simulink model "bf16_mac_new"  (R2022b)
settings: Solver=VariableStepAuto  StartTime=0.0  StopTime=10.0  RelTol=1e-3
libraries: hdlsllib x116, simulink x24
(part 2 of 2)

== system bf16_mac_new/bf16_adder/leading 2 ==
  u : Inport
  MATLAB Function : MATLAB Function  TreatAsAtomicUnit=on
  y : Outport
  wires:
  u/1 -> MATLAB Function/1(u)
  MATLAB Function/1(y) -> y/1

== system bf16_mac_new/bf16_adder/shift left1 ==
  In1 : Inport
  In2 : Inport  Port=2
  Constant : Constant  Value=2  OutDataTypeStr=half
  Data Type Conversion1 : DataTypeConversion  OutDataTypeStr=uint8  SaturateOnIntegerOverflow=off  RndMeth=Floor
  Data Type Conversion2 : DataTypeConversion  OutDataTypeStr=half  SaturateOnIntegerOverflow=off  RndMeth=Floor
  Pow : Math  Operator=pow  SignedPower=on  RndMeth=Zero
  Product : Product
  Out1 : Outport
  wires:
  Pow/1 -> Data Type Conversion1/1
  Constant/1 -> Pow/1
  In2/1 -> Data Type Conversion2/1
  Product/1 -> Out1/1
  Data Type Conversion1/1 -> Product/2
  Data Type Conversion2/1 -> Pow/2
  In1/1 -> Product/1

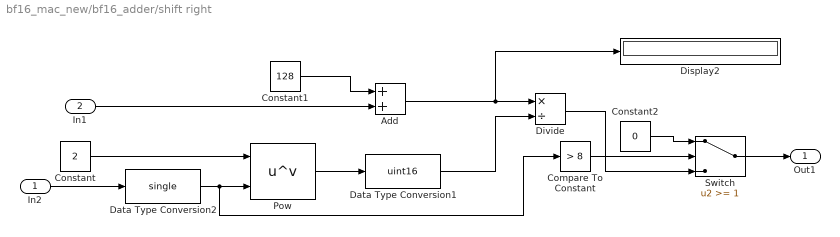
== system bf16_mac_new/bf16_adder/shift right ==
  In2 : Inport
  In1 : Inport  Port=2
  Add : Sum
  Compare To Constant : simulink/Logic and Bit Operations/Compare To Constant  relop=>  const=8  OutDataTypeStr=boolean
  Constant : Constant  Value=2  OutDataTypeStr=single
  Constant1 : Constant  Value=128  OutDataTypeStr=uint8
  Constant2 : Constant  Value=0  OutDataTypeStr=uint8
  Data Type Conversion1 : DataTypeConversion  OutDataTypeStr=uint16  SaturateOnIntegerOverflow=off  RndMeth=Floor
  Data Type Conversion2 : DataTypeConversion  OutDataTypeStr=single  SaturateOnIntegerOverflow=off  RndMeth=Floor
  Display2 : Display
      settings: Format=binary (Stored Integer)
  Divide : Product  Inputs=*/
  Pow : Math  Operator=pow  SignedPower=on  RndMeth=Zero
  Switch : Switch  Threshold=1  SaturateOnIntegerOverflow=off  InputSameDT=off
  Out1 : Outport
  wires:
  Pow/1 -> Data Type Conversion1/1
  Constant/1 -> Pow/1
  In2/1 -> Data Type Conversion2/1
  Data Type Conversion1/1 -> Divide/2
  Data Type Conversion2/1 -> Compare To Constant/1, Pow/2
  Add/1 -> Display2/1, Divide/1
  In1/1 -> Add/2
  Constant1/1 -> Add/1
  Compare To Constant/1 -> Switch/2
  Constant2/1 -> Switch/1
  Divide/1 -> Switch/3
  Switch/1 -> Out1/1

== system bf16_mac_new/bf16_adder/Multiplication1/bit slice ==
  Input : Inport
  Display : Display
      settings: Format=binary (Stored Integer)
  Extract Exponent : hdlsllib/Logic and Bit Operations/Bit Slice  lidx=14  ridx=7
  Extract Mantissa : hdlsllib/Logic and Bit Operations/Bit Slice  lidx=6  ridx=0
  Extract Sign : hdlsllib/Logic and Bit Operations/Bit Slice  lidx=15  ridx=15
  S1 : Outport
  E1 : Outport  Port=2
  M1 : Outport  Port=3
  wires:
  Input/1 -> Extract Mantissa/1, Extract Exponent/1, Extract Sign/1, Display/1
  Extract Mantissa/1 -> M1/1  "mantissa"
  Extract Sign/1 -> S1/1  "sign"
  Extract Exponent/1 -> E1/1

== system bf16_mac_new/bf16_adder/Multiplication1/bit slice1 ==
  Input : Inport
  Display : Display
      settings: Format=binary (Stored Integer)
  Extract Exponent : hdlsllib/Logic and Bit Operations/Bit Slice  lidx=14  ridx=7
  Extract Mantissa : hdlsllib/Logic and Bit Operations/Bit Slice  lidx=6  ridx=0
  Extract Sign : hdlsllib/Logic and Bit Operations/Bit Slice  lidx=15  ridx=15
  S2 : Outport
  E2 : Outport  Port=2
  M2 : Outport  Port=3
  wires:
  Input/1 -> Extract Mantissa/1, Extract Exponent/1, Extract Sign/1, Display/1
  Extract Mantissa/1 -> M2/1  "mantissa"
  Extract Sign/1 -> S2/1  "sign"
  Extract Exponent/1 -> E2/1

== system bf16_mac_new/bf16_adder/Subsystem3/bit slice ==
  Input : Inport
  Display : Display
      settings: Format=binary (Stored Integer)
  Extract Exponent : hdlsllib/Logic and Bit Operations/Bit Slice  lidx=14  ridx=7
  Extract Mantissa : hdlsllib/Logic and Bit Operations/Bit Slice  lidx=6  ridx=0
  Extract Sign : hdlsllib/Logic and Bit Operations/Bit Slice  lidx=15  ridx=15
  S1 : Outport
  E1 : Outport  Port=2
  M1 : Outport  Port=3
  wires:
  Input/1 -> Extract Mantissa/1, Extract Exponent/1, Extract Sign/1, Display/1
  Extract Mantissa/1 -> M1/1  "mantissa"
  Extract Sign/1 -> S1/1  "sign"
  Extract Exponent/1 -> E1/1

== system bf16_mac_new/bf16_adder/Subsystem3/bit slice1 ==
  Input : Inport
  Display : Display
      settings: Format=binary (Stored Integer)
  Extract Exponent : hdlsllib/Logic and Bit Operations/Bit Slice  lidx=14  ridx=7
  Extract Mantissa : hdlsllib/Logic and Bit Operations/Bit Slice  lidx=6  ridx=0
  Extract Sign : hdlsllib/Logic and Bit Operations/Bit Slice  lidx=15  ridx=15
  S2 : Outport
  E2 : Outport  Port=2
  M2 : Outport  Port=3
  wires:
  Input/1 -> Extract Mantissa/1, Extract Exponent/1, Extract Sign/1, Display/1
  Extract Mantissa/1 -> M2/1  "mantissa"
  Extract Sign/1 -> S2/1  "sign"
  Extract Exponent/1 -> E2/1

== system bf16_mac_new/bf16_adder/Subsystem3/leading 1 ==
  u : Inport
  MATLAB Function : MATLAB Function  TreatAsAtomicUnit=on
  y : Outport
  wires:
  u/1 -> MATLAB Function/1(u)
  MATLAB Function/1(y) -> y/1

== system bf16_mac_new/bf16_adder/Subsystem3/leading 2 ==
  u : Inport
  MATLAB Function : MATLAB Function  TreatAsAtomicUnit=on
  y : Outport
  wires:
  u/1 -> MATLAB Function/1(u)
  MATLAB Function/1(y) -> y/1

== system bf16_mac_new/bf16_adder/Subsystem3/shift left1 ==
  In1 : Inport
  In2 : Inport  Port=2
  Constant : Constant  Value=2  OutDataTypeStr=single  SampleTime=-1
  Data Type Conversion1 : DataTypeConversion  OutDataTypeStr=uint8  SaturateOnIntegerOverflow=off  RndMeth=Floor
  Data Type Conversion2 : DataTypeConversion  OutDataTypeStr=single  SaturateOnIntegerOverflow=off  RndMeth=Floor
  Pow : Math  Operator=pow  SignedPower=on  RndMeth=Zero
  Product : Product
  Out1 : Outport
  wires:
  Pow/1 -> Data Type Conversion1/1
  Constant/1 -> Pow/1
  In2/1 -> Data Type Conversion2/1
  Product/1 -> Out1/1
  Data Type Conversion1/1 -> Product/2
  Data Type Conversion2/1 -> Pow/2
  In1/1 -> Product/1

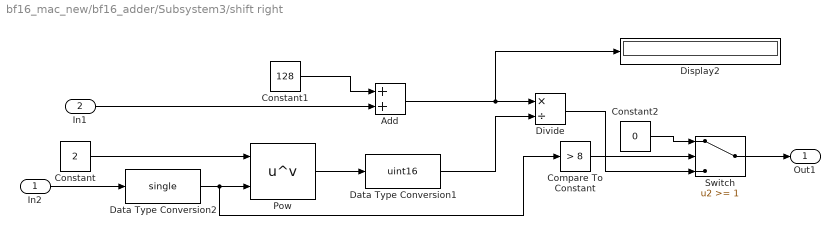
== system bf16_mac_new/bf16_adder/Subsystem3/shift right ==
  In2 : Inport
  In1 : Inport  Port=2
  Add : Sum
  Compare To Constant : simulink/Logic and Bit Operations/Compare To Constant  relop=>  const=8  OutDataTypeStr=boolean
  Constant : Constant  Value=2  OutDataTypeStr=single  SampleTime=-1
  Constant1 : Constant  Value=128  OutDataTypeStr=uint8  SampleTime=-1
  Constant2 : Constant  Value=0  OutDataTypeStr=uint8  SampleTime=-1
  Data Type Conversion1 : DataTypeConversion  OutDataTypeStr=uint16  SaturateOnIntegerOverflow=off  RndMeth=Floor
  Data Type Conversion2 : DataTypeConversion  OutDataTypeStr=single  SaturateOnIntegerOverflow=off  RndMeth=Floor
  Display2 : Display
      settings: Format=binary (Stored Integer)
  Divide : Product  Inputs=*/  RndMeth=Simplest  SaturateOnIntegerOverflow=on
  Pow : Math  Operator=pow  SignedPower=on  RndMeth=Zero
  Switch : Switch  Threshold=1  SaturateOnIntegerOverflow=off  InputSameDT=off
  Out1 : Outport
  wires:
  Pow/1 -> Data Type Conversion1/1
  Constant/1 -> Pow/1
  In2/1 -> Data Type Conversion2/1
  Data Type Conversion1/1 -> Divide/2
  Data Type Conversion2/1 -> Compare To Constant/1, Pow/2
  Add/1 -> Display2/1, Divide/1
  In1/1 -> Add/2
  Constant1/1 -> Add/1
  Compare To Constant/1 -> Switch/2
  Constant2/1 -> Switch/1
  Divide/1 -> Switch/3
  Switch/1 -> Out1/1

== matlab function bf16_mac_new/bf16_adder/leading 2/MATLAB Function ==
  data: u input; y output
function y = fcn(u)
v = double(u);
y = floor(log(v)/log(2));

== matlab function bf16_mac_new/MATLAB Function9 ==
  data: u input; y output
function y = fcn(u)
c = CustomFloat(u,16,7);
y = single(c);

== matlab function bf16_mac_new/MATLAB Function2 ==
  data: u input; y output
function y = fcn(u)
c = CustomFloat(u,16,7);
y = single(c);

== matlab function bf16_mac_new/MATLAB Function3 ==
  data: u input; y output
function y = fcn(u)

y = bitshift(u,16);

== matlab function bf16_mac_new/MATLAB Function ==
  data: u input; y output
function y = fcn(u)
c = CustomFloat(u,16,7);
y = single(c);

== matlab function bf16_mac_new/MATLAB Function4 ==
  data: u input; y output
function y = fcn(u)

y = bitshift(u,16);

== matlab function bf16_mac_new/MATLAB Function5 ==
  data: u input; y output
function y = fcn(u)
c = CustomFloat(u,16,7);
y = single(c);

== matlab function bf16_mac_new/MATLAB Function6 ==
  data: u input; y output
function y = fcn(u)

y = bitshift(u,16);

== matlab function bf16_mac_new/MATLAB Function7 ==
  data: u input; y output
function y = fcn(u)

y = bitshift(u,16);

== matlab function bf16_mac_new/accumulator/leading 1/MATLAB Function ==
  data: u input; y output
function y = fcn(u)
v = double(u);
y = floor(log(v)/log(2));

== matlab function bf16_mac_new/MATLAB Function1 ==
  data: u input; y output
function y = fcn(u)
c = CustomFloat(u,16,7);
y = single(c);

== matlab function bf16_mac_new/accumulator/leading 2/MATLAB Function ==
  data: u input; y output
function y = fcn(u)
v = double(u);
y = floor(log(v)/log(2));

== matlab function bf16_mac_new/bf16_adder/Subsystem3/leading 1/MATLAB Function ==
  data: u input; y output
function y = fcn(u)
v = double(u);
y = floor(log(v)/log(2));

== matlab function bf16_mac_new/MATLAB Function8 ==
  data: u input; y output
function y = fcn(u)

y = bitshift(u,16);

== matlab function bf16_mac_new/bf16_adder/leading 1/MATLAB Function ==
  data: u input; y output
function y = fcn(u)
v = double(u);
y = floor(log(v)/log(2));

== matlab function bf16_mac_new/bf16_adder/Subsystem3/leading 2/MATLAB Function ==
  data: u input; y output
function y = fcn(u)
v = double(u);
y = floor(log(v)/log(2));
